simulink model "manning_test_su_nonlinear"  (R2022b)
settings: Solver=VariableStepAuto  StartTime=0.0  StopTime=5*N  RelTol=1e-3
libraries: cstblocks x3
settings Model: Creator=chuan  LastModifiedBy=chuan

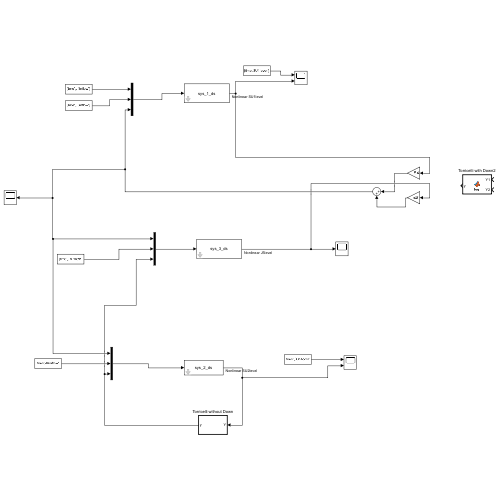
[thumbnail: Simulink's stored preview of the top-level diagram]
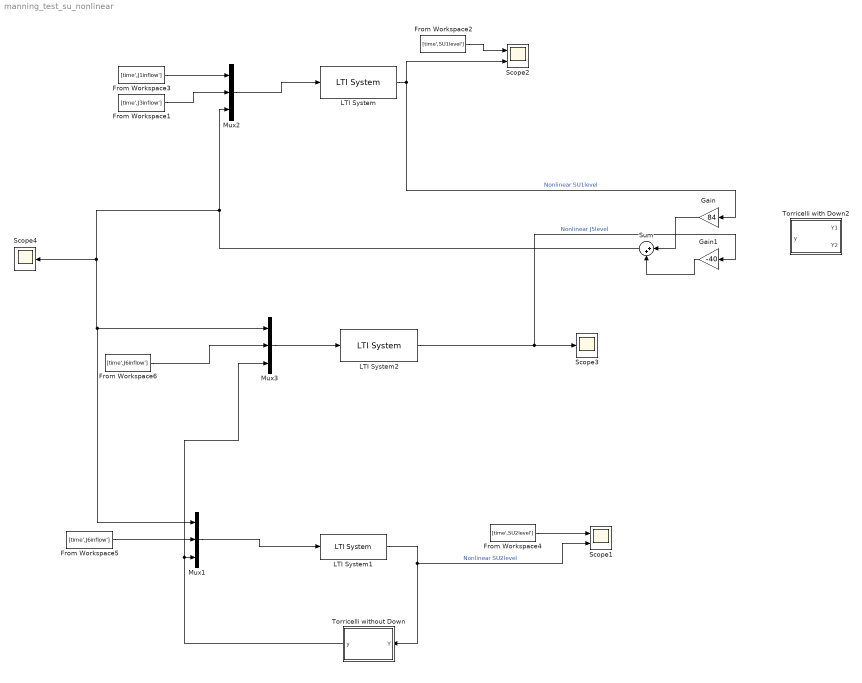
== system manning_test_su_nonlinear ==
  From Workspace1 : FromWorkspace  VariableName=[time',J3inflow']
  From Workspace2 : FromWorkspace  VariableName=[time',SU1level']
  From Workspace3 : FromWorkspace  VariableName=[time',J1inflow']
  From Workspace4 : FromWorkspace  VariableName=[time',SU2level']
  From Workspace5 : FromWorkspace  VariableName=[time',J6inflow']
  From Workspace6 : FromWorkspace  VariableName=[time',J6inflow']
  Gain : Gain  Gain=84
  Gain1 : Gain  Gain=-40
  LTI System : cstblocks/LTI System  sys=sys_1_ds  IC=[]
  LTI System1 : cstblocks/LTI System  sys=sys_2_ds  IC=[]
  LTI System2 : cstblocks/LTI System  sys=sys_3_ds  IC=[]
  Mux1 : Mux  Inputs=3
  Mux2 : Mux  Inputs=3
  Mux3 : Mux  Inputs=3
  Scope1 : Scope  NumInputPorts=2
  Scope2 : Scope  NumInputPorts=2
  Scope3 : Scope
  Scope4 : Scope
  Sum : Sum  Inputs=|++
  Torricelli with Down2 : MATLAB Function  TreatAsAtomicUnit=on
  Torricelli without Down : MATLAB Function  TreatAsAtomicUnit=on
  wires:
  LTI System/1 -> Gain/1, Scope2/2  "Nonlinear SU1level"
  From Workspace3/1 -> Mux2/1
  From Workspace1/1 -> Mux2/2
  Mux2/1 -> LTI System/1
  From Workspace2/1 -> Scope2/1
  LTI System1/1 -> Scope1/2, Torricelli without Down/1(Y)  "Nonlinear SU2level"
  From Workspace4/1 -> Scope1/1
  Torricelli without Down/1(y) -> Mux3/3, Mux1/3
  Mux1/1 -> LTI System1/1
  Sum/1 -> Scope4/1, Mux1/1, Mux3/1, Mux2/3
  From Workspace6/1 -> Mux3/2
  LTI System2/1 -> Gain1/1, Scope3/1  "Nonlinear J5level"
  Mux3/1 -> LTI System2/1
  From Workspace5/1 -> Mux1/2
  Gain/1 -> Sum/1
  Gain1/1 -> Sum/2

== matlab function manning_test_su_nonlinear/Torricelli with Down2 ==
  data: Y1 input; y output; Y2 input
function y = fcn(Y1,Y2)
Cd = 0.65;
A0 = 144;
g = 9.81;
Z0 = 9;
Yfull = 12;
H_star = Z0 + Yfull;

Y1 = max(Y1,0);
Y2 = max(Y2,0);
H1 = Y1 + Z0;
H2 = Y2 + Z0;

if H1 >= H_star
    if H2 <= Z0 + Yfull/2
        He = H1 - (Z0 + Yfull/2);
    else
        He = H1-H2;
    end
   

    if He >= 0
        y = Cd*A0*sqrt(2*g*He);
    else
        y = -Cd*A0*sqrt(2*g*-He);
    end
else
    CwL = (Cd*A0*sqrt(g))/(Yfull);
    y = CwL*(H1-Z0)^(1.5);
    
end

== matlab function manning_test_su_nonlinear/Torricelli without Down ==
  data: Y input; y output
function y = fcn(Y)
Cd = 0.65;
A0 = 324;
g = 9.81;
Z0 = 2.2;
Yfull = 18;
H_star = Z0 + Yfull;

Y = max(Y,0);
H1 = Y + Z0;

if H1 >= H_star
    He = H1 - (Z0 + Yfull/2);
    y = Cd*A0*sqrt(2*g*He);
else
    CwL = (Cd*A0*sqrt(g))/(Yfull);
    y = CwL*(H1-Z0)^(1.5);
end
